simulink model "MAIN_FILE"  (R2023a)
settings: Solver=VariableStepAuto  StartTime=0.0  StopTime=2  RelTol=1e-3
libraries: simulink x6, fuzblock x4, spsVoltageMeasurementLib x3, spsControlledVoltageSourceLib x1, spsPermanentMagnetSynchronousMachineLib x1, spsUniversalBridgeLib x1, spspowerguiLib x1
settings Model: SimulationMode=accelerator  Creator=malif  LastModifiedBy=malif
settings ModelReferenceCC: EnableRefExpFcnMdlSchedulingChecks=on

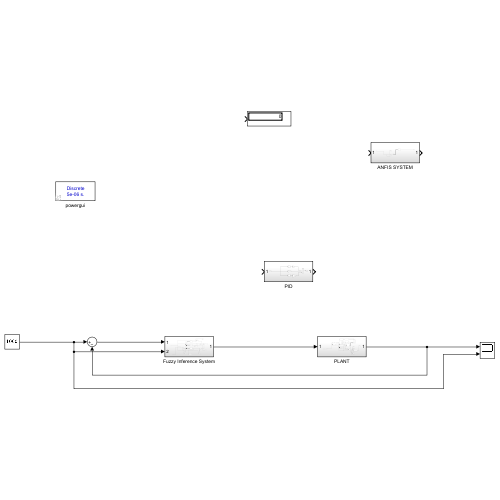
[thumbnail: Simulink's stored preview of the top-level diagram]
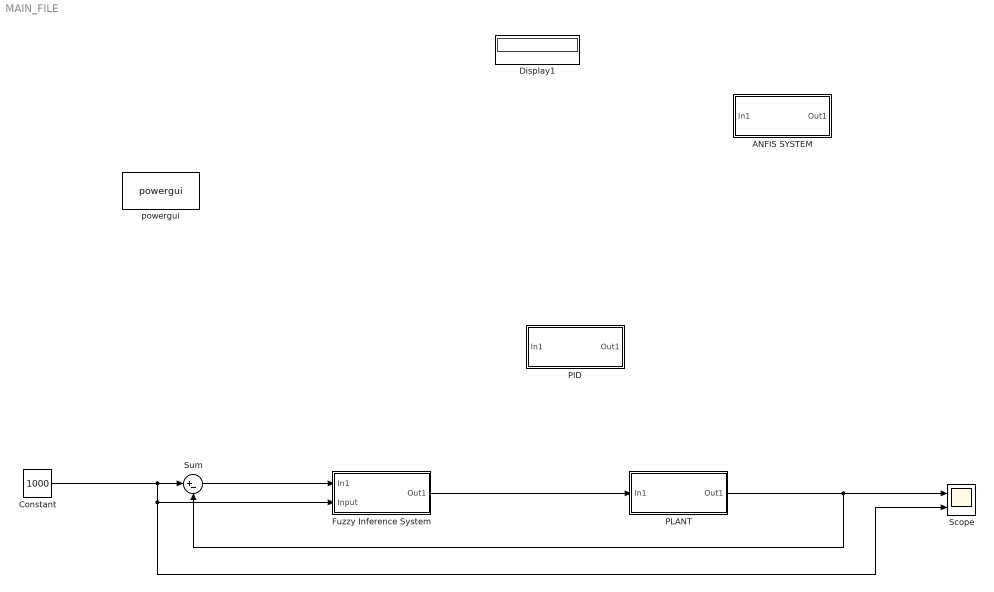
== system MAIN_FILE ==
  ANFIS SYSTEM : Subsystem
  Constant : Constant  Value=1000
  Display1 : Display
  Fuzzy Inference System : Subsystem
  PID : Subsystem
  PLANT : Subsystem
  Scope : Scope  NumInputPorts=2
  Sum : Sum  Inputs=|+-
  powergui : spspowerguiLib/powergui  Priority=1  SimulationMode=Discrete  SampleTime=5e-6  frequency=60  Iterations=50  frequencyindice=0  Pbase=100e6  ErrMax=1e-4  UnitsV=kV  UnitsW=MW  buscounter=0  FunctionMessages=off  echomessages=off  EnableUseOfTLC=off  CurrentSourceSwitches=off  DisableSnubberDevices=off  DisableRonSwitches=off  DisableVfSwitches=off  DisplayEquations=off  AutomaticDiscreteSolvers=off  SolverType=Tustin/Backward Euler (TBE)  Interpol=off  ExternalGateDelay=off  methode=off  Ts=100  x0status=blocks  SPID=on  SwTol=0  HookPort=off  NonlinearTolerance=1e-4  nMaxIteration=100  ContinueOnMaxIteration=off  RestoreLinks=warning  ResistiveCurrentMeasurement=off  Frange=[0:2:500]  Ylog=off  Xlog=on  ShowGrid=off  save=off  variable=ZData  structure=0  ZoomFFT=off  StartTime=0.0  cycles=1  DisplayStyle=1  fundamental=60  FreqAxis=off  MaxFrequency=1000  frequencyindicesteady=1  RmsSteady=1  display=off
  wires:
  Constant/1 -> Fuzzy Inference System/2(Input), Scope/2, Sum/1
  PLANT/1(Out1) -> Scope/1, Sum/2
  Fuzzy Inference System/1(Out1) -> PLANT/1(In1)
  Sum/1 -> Fuzzy Inference System/1(In1)

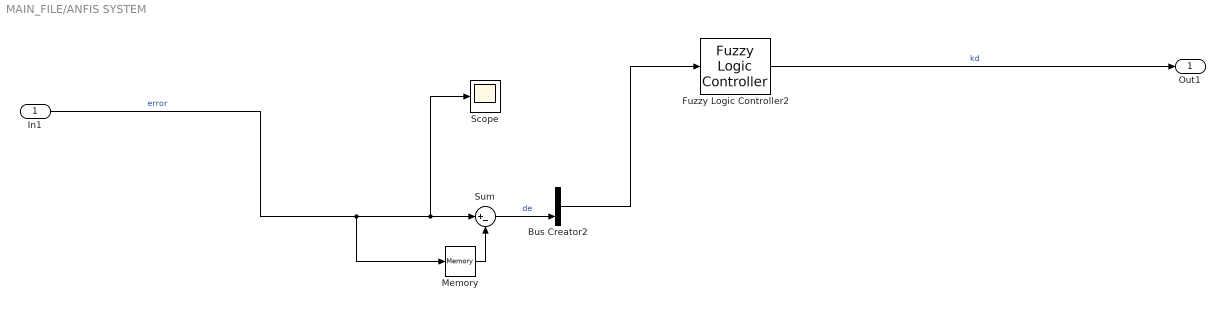
== system MAIN_FILE/ANFIS SYSTEM ==
  In1 : Inport
  Bus Creator2 : BusCreator  Inputs=2
  Fuzzy Logic Controller2 : fuzblock/Fuzzy Logic  Controller  FIS='neurofis.fis'  OutputSampleNumber=101  DataType=double  FuzzifiedInputs=off  RuleFiringStrengths=off  RuleOutputs=off  AggregatedOutputs=off  SimulateUsing=Code generation  OutOfRangeInputValueMessage=warning  NoRuleFiredMessage=warning  EmptyOutputFuzzySetMessage=warning
  Memory : Memory  LinearizeMemory=on  LinearizeAsDelay=on
  Scope : Scope
  Sum : Sum  Inputs=|+-
  Out1 : Outport
  wires:
  In1/1 -> Memory/1, Scope/1, Sum/1  "error"
  Bus Creator2/1 -> Fuzzy Logic Controller2/1
  Memory/1 -> Sum/2
  Sum/1 -> Bus Creator2/2  "de"
  Fuzzy Logic Controller2/1 -> Out1/1  "kd"

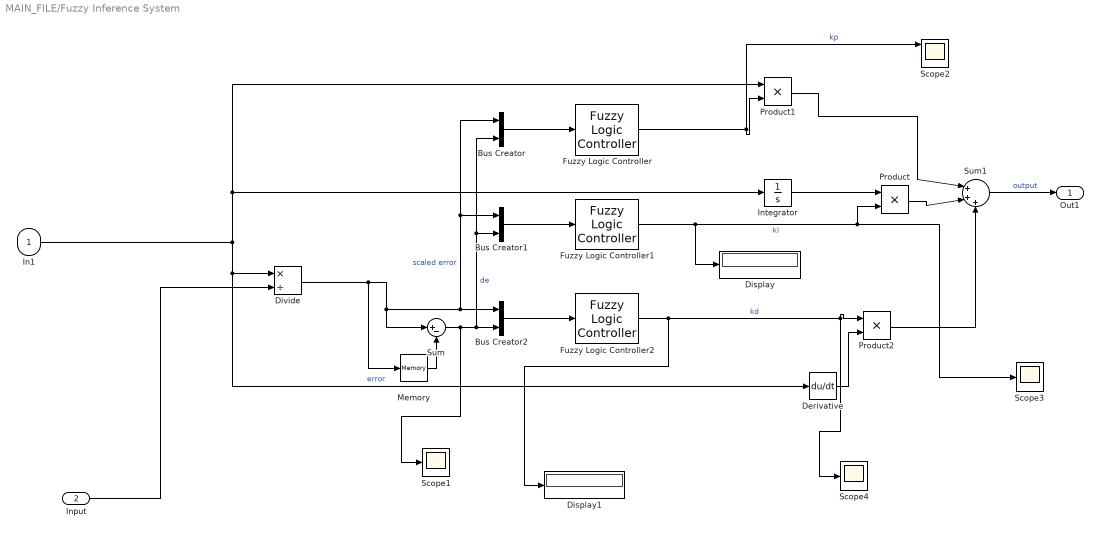
== system MAIN_FILE/Fuzzy Inference System ==
  In1 : Inport
  Input : Inport  Port=2
  Bus Creator : BusCreator  Inputs=2
  Bus Creator1 : BusCreator  Inputs=2
  Bus Creator2 : BusCreator  Inputs=2
  Derivative : Derivative
  Display : Display
  Display1 : Display
  Divide : Product  Inputs=*/
  Fuzzy Logic Controller : fuzblock/Fuzzy Logic  Controller  FIS='kp_fuzzy2.fis'  OutputSampleNumber=101  DataType=double  FuzzifiedInputs=off  RuleFiringStrengths=off  RuleOutputs=off  AggregatedOutputs=off  SimulateUsing=Interpreted execution  OutOfRangeInputValueMessage=warning  NoRuleFiredMessage=warning  EmptyOutputFuzzySetMessage=warning
  Fuzzy Logic Controller1 : fuzblock/Fuzzy Logic  Controller  FIS='ki_fuzzy2.fis'  OutputSampleNumber=101  DataType=double  FuzzifiedInputs=off  RuleFiringStrengths=off  RuleOutputs=off  AggregatedOutputs=off  SimulateUsing=Code generation  OutOfRangeInputValueMessage=warning  NoRuleFiredMessage=warning  EmptyOutputFuzzySetMessage=warning
  Fuzzy Logic Controller2 : fuzblock/Fuzzy Logic  Controller  FIS='kd_fuzzy2.fis'  OutputSampleNumber=101  DataType=double  FuzzifiedInputs=off  RuleFiringStrengths=off  RuleOutputs=off  AggregatedOutputs=off  SimulateUsing=Code generation  OutOfRangeInputValueMessage=warning  NoRuleFiredMessage=warning  EmptyOutputFuzzySetMessage=warning
  Integrator : Integrator
  Memory : Memory  LinearizeMemory=on  LinearizeAsDelay=on
  Product : Product
  Product1 : Product
  Product2 : Product
  Scope1 : Scope
  Scope2 : Scope  NumInputPorts=3
  Scope3 : Scope
  Scope4 : Scope
  Sum : Sum  Inputs=|+-
  Sum1 : Sum  Inputs=|+++
  Out1 : Outport
  wires:
  Bus Creator/1 -> Fuzzy Logic Controller/1
  Bus Creator1/1 -> Fuzzy Logic Controller1/1
  Bus Creator2/1 -> Fuzzy Logic Controller2/1
  Fuzzy Logic Controller/1 -> Product1/2, Scope2/1  "kp"
  Fuzzy Logic Controller1/1 -> Product/2, Scope3/1, Display/1  "ki"
  Fuzzy Logic Controller2/1 -> Product2/1, Scope4/1, Display1/1  "kd"
  Memory/1 -> Sum/2
  Sum/1 -> Scope1/1, Bus Creator/2, Bus Creator1/2, Bus Creator2/2  "de"
  Integrator/1 -> Product/1
  Derivative/1 -> Product2/2
  Product/1 -> Sum1/2
  Sum1/1 -> Out1/1  "output"
  In1/1 -> Divide/1, Derivative/1, Integrator/1, Product1/1  "error"
  Product1/1 -> Sum1/1
  Product2/1 -> Sum1/3
  Input/1 -> Divide/2
  Divide/1 -> Memory/1, Bus Creator/1, Bus Creator1/1, Bus Creator2/1, Sum/1  "scaled error"

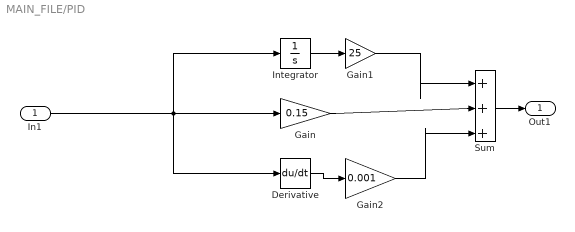
== system MAIN_FILE/PID ==
  In1 : Inport
  Derivative : Derivative
  Gain : Gain  Gain=0.15
  Gain1 : Gain  Gain=25
  Gain2 : Gain  Gain=0.001
  Integrator : Integrator
  Sum : Sum  Inputs=|+++
  Out1 : Outport
  wires:
  Sum/1 -> Out1/1
  Derivative/1 -> Gain2/1
  Integrator/1 -> Gain1/1
  In1/1 -> Derivative/1, Integrator/1, Gain/1
  Gain1/1 -> Sum/1
  Gain2/1 -> Sum/3
  Gain/1 -> Sum/2

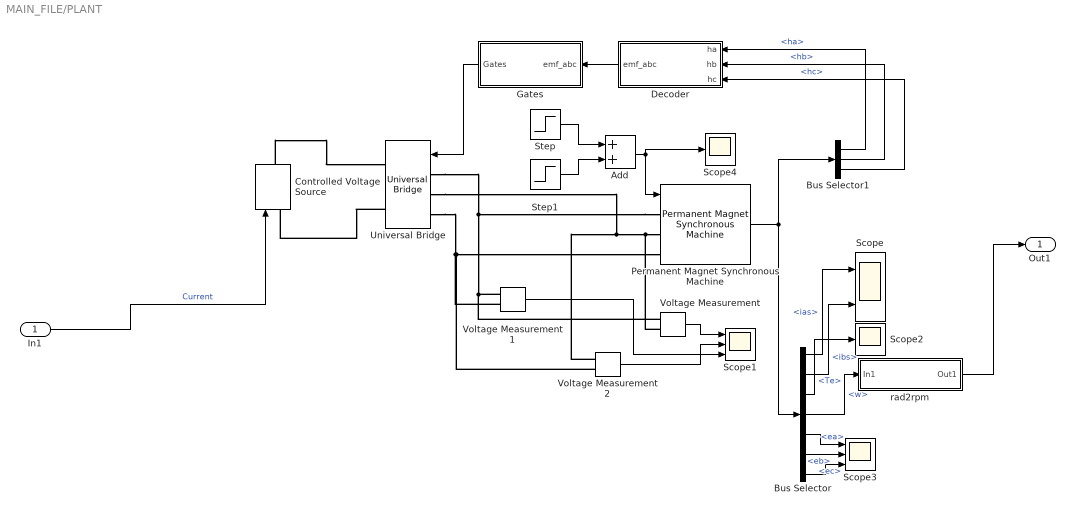
== system MAIN_FILE/PLANT ==
  In1 : Inport
  Add : Sum
  Bus Selector : BusSelector  OutputSignals=ias,ibs,Te,w,ea,eb,ec
  Bus Selector1 : BusSelector  OutputSignals=ha,hb,hc
  Controlled Voltage Source : spsControlledVoltageSourceLib/Controlled Voltage Source  Initialize=on  Source_Type=DC  Amplitude=0  Phase=0  Frequency=0  Measurements=None
  Decoder : Subsystem
  Gates : Subsystem
  Permanent Magnet Synchronous Machine : spsPermanentMagnetSynchronousMachineLib/Permanent Magnet Synchronous Machine  NbPhases=3  FluxDistribution=Trapezoidal  RotorType=Round  MechanicalLoad=Torque Tm  PresetModel=No  ShowDetailedParameters=on  MeasurementBus=on  Resistance=0.0485  Inductance=8.5e-3  dqInductances=[8.5e-3,8.5e-3]  La=0.000395  MachineConstant=Flux linkage established by magnets (V.s)  Flux=0.1194  VoltageCst=100.0283  TorqueCst=0.9552  Flat=120  Mechanical=[0.0027 0.0004924 4 0]  PolePairs=4  InitialConditions=[0,0, 0,0]  InitialConditions5ph=[0 0 0 0 0 0]  RefAngle=90 degrees behind phase A axis (modified Park)  IterativeDiscreteModel=Trapezoidal non iterative  TsBlock=-1  TsPowergui=0
  Scope : Scope  NumInputPorts=2
  Scope1 : Scope  NumInputPorts=3
  Scope2 : Scope
  Scope3 : Scope  NumInputPorts=3
  Scope4 : Scope
  Step : Step  Time=0.75  Before=10  After=20  SampleTime=0
  Step1 : Step  Time=1.5  After=-5  SampleTime=0
  Universal Bridge : spsUniversalBridgeLib/Universal Bridge  Arms=3  SnubberResistance=1e5  SnubberCapacitance=inf  Device=MOSFET / Diodes  Ron=1e-3  Lon=0  ForwardVoltages="[  0  0  ]"  ForwardVoltage=0  GTOparameters=[ 10e-6 , 20e-6 ]  IGBTparameters=[ 1e-6 , 2e-6 ]  Measurements=None  Measurements_2=None  converterType=Rectifier
  Voltage Measurement : spsVoltageMeasurementLib/Voltage Measurement  PhasorSimulation=off  OutputType=Complex  PSBequivalent=0
  Voltage Measurement1 : spsVoltageMeasurementLib/Voltage Measurement  PhasorSimulation=off  OutputType=Complex  PSBequivalent=0
  Voltage Measurement2 : spsVoltageMeasurementLib/Voltage Measurement  PhasorSimulation=off  OutputType=Complex  PSBequivalent=0
  rad2rpm : Subsystem
  Out1 : Outport
  wires:
  Bus Selector/2 -> Scope/2  "<ibs>"
  Bus Selector/1 -> Scope/1  "<ias>"
  Permanent Magnet Synchronous Machine/1 -> Bus Selector1/1, Bus Selector/1
  Voltage Measurement/1 -> Scope1/1
  Bus Selector/4 -> rad2rpm/1(In1)  "<w>"
  rad2rpm/1(Out1) -> Out1/1
  In1/1 -> Controlled Voltage Source/1  "Current"
  Voltage Measurement1/1 -> Scope1/3
  Gates/1(Gates) -> Universal Bridge/1
  Decoder/1(emf_abc) -> Gates/1(emf_abc)
  Bus Selector1/3 -> Decoder/3(hc)  "<hc>"
  Bus Selector1/2 -> Decoder/2(hb)  "<hb>"
  Bus Selector1/1 -> Decoder/1(ha)  "<ha>"
  Voltage Measurement2/1 -> Scope1/2
  Bus Selector/3 -> Scope2/1  "<Te>"
  Bus Selector/5 -> Scope3/1  "<ea>"
  Bus Selector/6 -> Scope3/2  "<eb>"
  Bus Selector/7 -> Scope3/3  "<ec>"
  Step/1 -> Add/1
  Step1/1 -> Add/2
  Add/1 -> Permanent Magnet Synchronous Machine/1, Scope4/1
  connections:
  Permanent Magnet Synchronous Machine/LConn1 -- Universal Bridge/LConn1 -- Voltage Measurement1/LConn1 -- Voltage Measurement/LConn1
  Permanent Magnet Synchronous Machine/LConn3 -- Voltage Measurement2/LConn2 -- Universal Bridge/LConn3 -- Voltage Measurement1/LConn2
  Voltage Measurement/LConn2 -- Universal Bridge/LConn2 -- Voltage Measurement2/LConn1 -- Permanent Magnet Synchronous Machine/LConn2
  Universal Bridge/RConn2 -- Controlled Voltage Source/LConn1
  Controlled Voltage Source/RConn1 -- Universal Bridge/RConn1

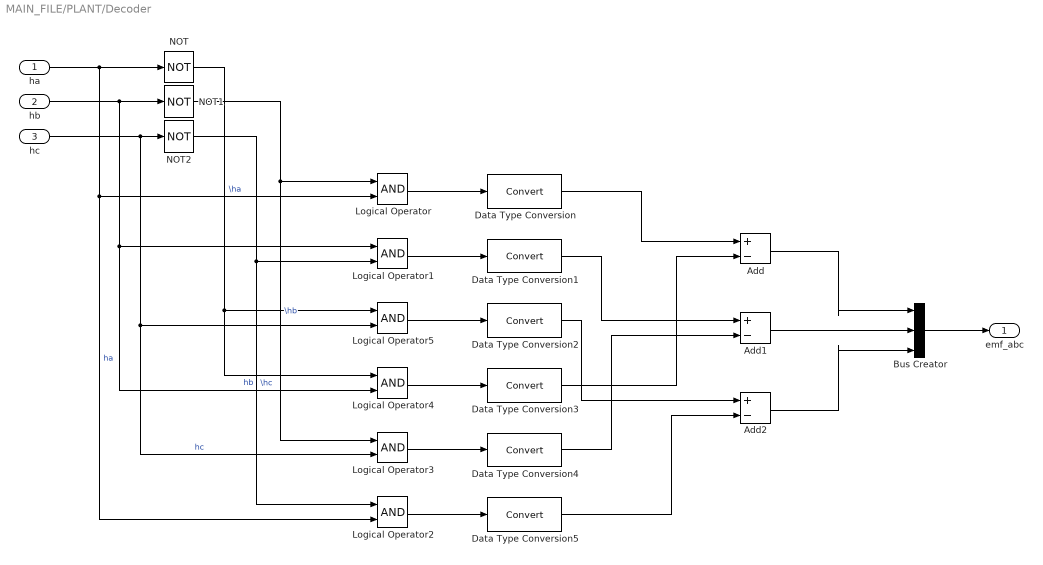
== system MAIN_FILE/PLANT/Decoder ==
  ha : Inport
  hb : Inport  Port=2
  hc : Inport  Port=3
  Add : Sum  Inputs=+-
  Add1 : Sum  Inputs=+-
  Add2 : Sum  Inputs=+-
  Bus Creator : BusCreator  Inputs=3
  Data Type Conversion{,1..5} (6 alike) : DataTypeConversion  SaturateOnIntegerOverflow=off  RndMeth=Floor
  Logical Operator{,1..5} (6 alike) : Logic  AllPortsSameDT=off  OutDataTypeStr=boolean
  NOT : Logic  Operator=NOT  IconShape=distinctive  AllPortsSameDT=off  OutDataTypeStr=boolean
  NOT1 : Logic  Operator=NOT  IconShape=distinctive  AllPortsSameDT=off  OutDataTypeStr=boolean
  NOT2 : Logic  Operator=NOT  IconShape=distinctive  AllPortsSameDT=off  OutDataTypeStr=boolean
  emf_abc : Outport
  wires:
  ha/1 -> Logical Operator2/2, Logical Operator/2, NOT/1  "ha"
  hb/1 -> Logical Operator4/2, Logical Operator1/1, NOT1/1  "hb"
  NOT1/1 -> Logical Operator3/1, Logical Operator/1  "\\hb"
  NOT2/1 -> Logical Operator2/1, Logical Operator1/2  "\\hc"
  hc/1 -> Logical Operator3/2, Logical Operator5/2, NOT2/1  "hc"
  NOT/1 -> Logical Operator4/1, Logical Operator5/1  "\\ha"
  Logical Operator/1 -> Data Type Conversion/1
  Logical Operator1/1 -> Data Type Conversion1/1
  Logical Operator5/1 -> Data Type Conversion2/1
  Logical Operator4/1 -> Data Type Conversion3/1
  Logical Operator3/1 -> Data Type Conversion4/1
  Logical Operator2/1 -> Data Type Conversion5/1
  Data Type Conversion/1 -> Add/1
  Data Type Conversion3/1 -> Add/2
  Data Type Conversion1/1 -> Add1/1
  Data Type Conversion4/1 -> Add1/2
  Data Type Conversion2/1 -> Add2/1
  Data Type Conversion5/1 -> Add2/2
  Add/1 -> Bus Creator/1
  Add1/1 -> Bus Creator/2
  Add2/1 -> Bus Creator/3
  Bus Creator/1 -> emf_abc/1

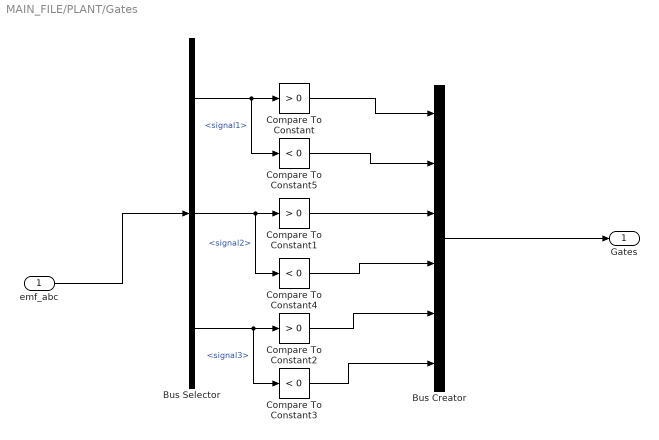
== system MAIN_FILE/PLANT/Gates ==
  emf_abc : Inport
  Bus Creator : BusCreator  Inputs=6
  Bus Selector : BusSelector  OutputSignals=signal1,signal2,signal3
  Compare To Constant : simulink/Logic and Bit Operations/Compare To Constant  relop=>  const=0  OutDataTypeStr=boolean
  Compare To Constant1 : simulink/Logic and Bit Operations/Compare To Constant  relop=>  const=0  OutDataTypeStr=boolean
  Compare To Constant2 : simulink/Logic and Bit Operations/Compare To Constant  relop=>  const=0  OutDataTypeStr=boolean
  Compare To Constant3 : simulink/Logic and Bit Operations/Compare To Constant  relop=<  const=0  OutDataTypeStr=boolean
  Compare To Constant4 : simulink/Logic and Bit Operations/Compare To Constant  relop=<  const=0  OutDataTypeStr=boolean
  Compare To Constant5 : simulink/Logic and Bit Operations/Compare To Constant  relop=<  const=0  OutDataTypeStr=boolean
  Gates : Outport
  wires:
  emf_abc/1 -> Bus Selector/1
  Bus Selector/1 -> Compare To Constant5/1, Compare To Constant/1  "<signal1>"
  Bus Selector/2 -> Compare To Constant4/1, Compare To Constant1/1  "<signal2>"
  Bus Selector/3 -> Compare To Constant3/1, Compare To Constant2/1  "<signal3>"
  Compare To Constant/1 -> Bus Creator/1
  Compare To Constant5/1 -> Bus Creator/2
  Compare To Constant1/1 -> Bus Creator/3
  Compare To Constant4/1 -> Bus Creator/4
  Compare To Constant2/1 -> Bus Creator/5
  Compare To Constant3/1 -> Bus Creator/6
  Bus Creator/1 -> Gates/1

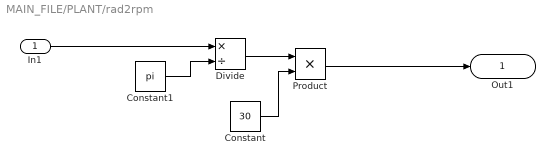
== system MAIN_FILE/PLANT/rad2rpm ==
  In1 : Inport
  Constant : Constant  Value=30
  Constant1 : Constant  Value=pi
  Divide : Product  Inputs=*/
  Product : Product
  Out1 : Outport
  wires:
  In1/1 -> Divide/1
  Divide/1 -> Product/1
  Constant1/1 -> Divide/2
  Constant/1 -> Product/2
  Product/1 -> Out1/1
